simulink model "TankSimplesNEW"  (R2016a)
settings: Solver=VariableStepAuto  StartTime=0.0  StopTime=20  RelTol=1e-3
settings Model: Creator=Ítalo Renan  LastModifiedBy=Ítalo Renan

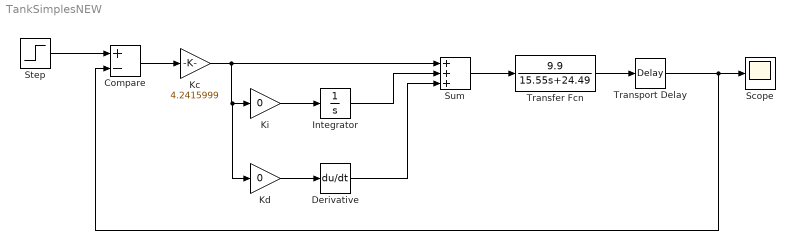
== system TankSimplesNEW ==
  Compare : Sum  Inputs=+-
  Derivative : Derivative
  Integrator : Integrator
  Kc : Gain  Gain=4.2415999
  Kd : Gain  Gain=0
  Ki : Gain  Gain=0
  Scope : Scope
  Step : Step  After=15  SampleTime=0.01
  Sum : Sum  Inputs=3
  Transfer Fcn : TransferFcn  Numerator=[9.9]  Denominator=[15.55 24.49]
  Transport Delay : TransportDelay
  wires:
  Ki/1 -> Integrator/1
  Kd/1 -> Derivative/1
  Step/1 -> Compare/1
  Kc/1 -> Sum/1, Kd/1, Ki/1
  Integrator/1 -> Sum/2
  Derivative/1 -> Sum/3
  Transfer Fcn/1 -> Transport Delay/1
  Transport Delay/1 -> Compare/2, Scope/1
  Sum/1 -> Transfer Fcn/1
  Compare/1 -> Kc/1
